simulink subsystem "LRLM_ECU_V6"  (R2021a)
settings: Solver=VariableStepAuto  StartTime=0.0  StopTime=10.0  RelTol=1e-3
libraries: LRLM x6
settings Model: Creator=Sai229  LastModifiedBy=Sai229

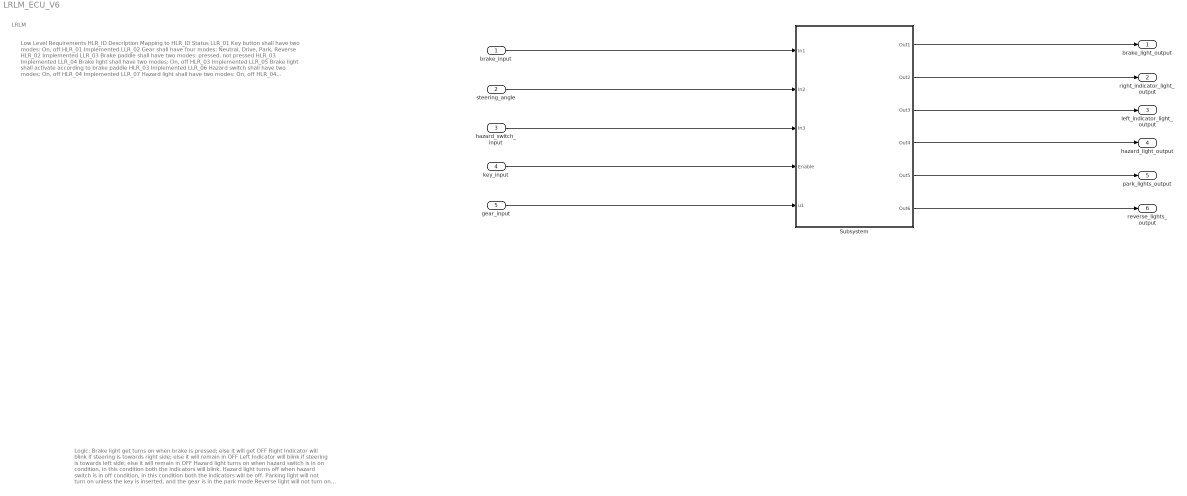
== system LRLM_ECU_V6 ==
  note: Low Level Requirements
      |
      | HLR_ID
      | Description
      | Mapping to HLR_ID
      | Status
      |
      | LLR_01
      | Key button shall have two modes: On, off
      | HLR_01
      | Implemented
      |
      | LLR_02
      | Gear shall have four modes: Neutral, Drive, Park, Reverse
      | HLR_02
      | Implemented
      |
      | LLR_03
      | Brake paddle shall have two modes: pressed, not pressed
      | HLR_03
      | Implemented
      |
      | LLR_04
      | Brake light shall have two modes: On, off
      | HLR_03
      | Implemented
      |
      | LLR_05
      | Brake light shall activate according to brake paddle
      | HLR_03
      | Implemented
      |
      | LLR_06
      | Hazard switch shall have two modes: On, off
      | HLR_04
      | Implemented
      |
      | LLR_07
      | Hazard light shall have two modes: On, off
      | HLR_04
      | Implemented
      |
      | LLR_08
      | Hazard light shall activate according to hazard switch
      | HLR_04
      | Implemented
      |
      | LLR_09
      | Steering shall move in both the directions
      | HLR_05
      | Implemented
      |
      | LLR_10
      | Right Indicator light shall have two modes: On, off
      | HLR_05
      | Implemented
      |
      | LLR_11
      | Left Indicator light shall have two modes: On, off
      | HLR_05
      | Implemented
      |
      | LLR_12
      | Right indicator light shall activate according to steering angle
      | HLR_05
      | Implemented
      |
      | LLR_13
      | Left indicator light shall activate according to steering angle
      | HLR_05
      | Implemented
      |
      | LLR_14
      | Park light shall have two modes: On, off
      | HLR_06
      | Implemented
      |
      | LLR_15
      | Parking light shall activate according to park gear and key button
      | HLR_06
      | Implemented
      |
      | LLR_16
      | Reverse light shall have two modes: On, off
      | HLR_07
      | Implemented
      |
      | LLR_17
      | Reversing lights shall activate according to reverse gear and key button
      | HLR_07
      | Implemented
  note: Logic:
      | Brake light get turns on when brake is pressed; else it will get OFF
      | Right Indicator will blink if steering is towards right side; else it will remain in OFF
      | Left Indicator will blink if steering is towards left side; else it will remain in OFF
      | Hazard light turns on when hazard switch is in on condition, in this condition both the indicators will blink.
      | Hazard light turns off when hazard switch is in off condition, in this condition both the indicators will be off.
      | Parking light will not turn on unless the key is inserted, and the gear is in the park mode
      | Reverse light will not turn on unless the key is inserted, and the gear is in the reverse mode
  note: LRLM
  brake_input : Inport
  steering_angle : Inport  Port=2
  hazard_switch_input : Inport  Port=3
  key_input : Inport  Port=4
  gear_input : Inport  Port=5
  Subsystem : Subsystem
  brake_light_output : Outport
  right_indicator_light_output : Outport  Port=2
  left_indicator_light_output : Outport  Port=3
  hazard_light_output : Outport  Port=4
  park_lights_output : Outport  Port=5
  reverse_lights_output : Outport  Port=6
  wires:
  brake_input/1 -> Subsystem/1(In1)
  steering_angle/1 -> Subsystem/2(In2)
  hazard_switch_input/1 -> Subsystem/3(In3)
  key_input/1 -> Subsystem/4(Enable)
  gear_input/1 -> Subsystem/5(u1)
  Subsystem/1(Out1) -> brake_light_output/1
  Subsystem/2(Out2) -> right_indicator_light_output/1
  Subsystem/3(Out3) -> left_indicator_light_output/1
  Subsystem/4(Out4) -> hazard_light_output/1
  Subsystem/5(Out5) -> park_lights_output/1
  Subsystem/6(Out6) -> reverse_lights_output/1

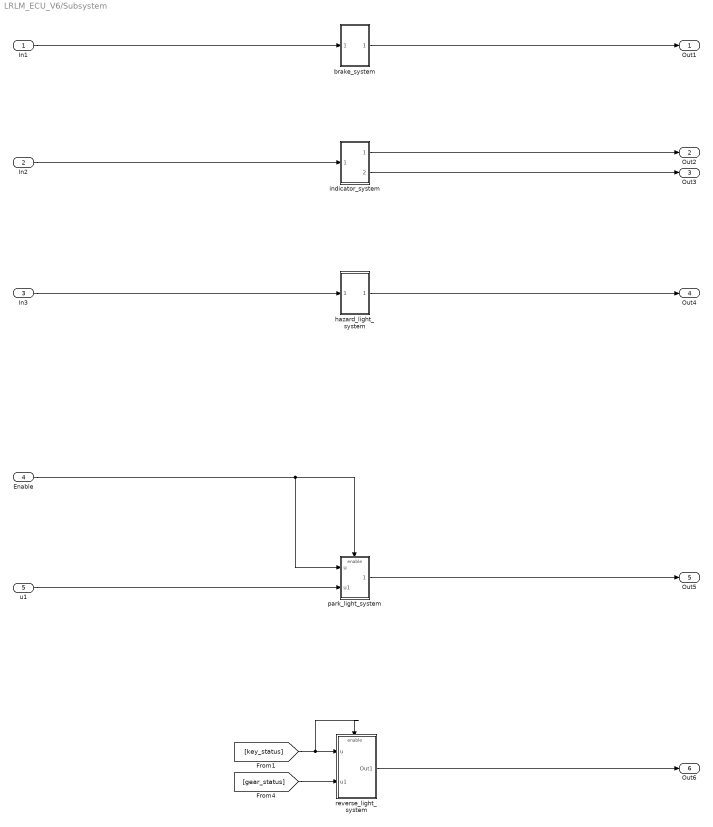
== system LRLM_ECU_V6/Subsystem ==
  In1 : Inport
  In2 : Inport  Port=2
  In3 : Inport  Port=3
  Enable : Inport  Port=4
  u1 : Inport  Port=5
  brake_system : Subsystem
  hazard_light_system : Subsystem
  indicator_system : Subsystem
  park_light_system : Subsystem
  reverse_light_system : Subsystem
  Out1 : Outport
  Out2 : Outport  Port=2
  Out3 : Outport  Port=3
  Out4 : Outport  Port=4
  Out5 : Outport  Port=5
  Out6 : Outport  Port=6
  wires:
  In3/1 -> hazard_light_system/1(In1)
  [gear_status] -> reverse_light_system/2(u1)
  hazard_light_system/1(Out1) -> Out4/1
  park_light_system/1(Out1) -> Out5/1
  [key_status] -> reverse_light_system/1(u), reverse_light_system/Enable
  Enable/1 -> park_light_system/Enable, park_light_system/1(u)
  indicator_system/2(Out2) -> Out3/1
  In2/1 -> indicator_system/1(In1)
  In1/1 -> brake_system/1(In1)
  indicator_system/1(Out1) -> Out2/1
  reverse_light_system/1(Out1) -> Out6/1
  u1/1 -> park_light_system/2(u1)
  brake_system/1(Out1) -> Out1/1

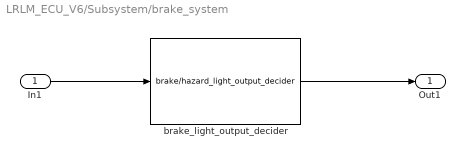
== system LRLM_ECU_V6/Subsystem/brake_system ==
  In1 : Inport
  brake_light_output_decider : LRLM/brake//hazard_light_output_decider
      settings: SourceProductName=LRLM Library
  Out1 : Outport
  wires:
  brake_light_output_decider/1 -> Out1/1
  In1/1 -> brake_light_output_decider/1

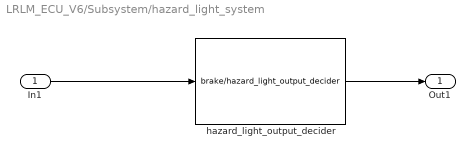
== system LRLM_ECU_V6/Subsystem/hazard_light_system ==
  In1 : Inport
  hazard_light_output_decider : LRLM/brake//hazard_light_output_decider
      settings: SourceProductName=LRLM Library
  Out1 : Outport
  wires:
  hazard_light_output_decider/1 -> Out1/1
  In1/1 -> hazard_light_output_decider/1

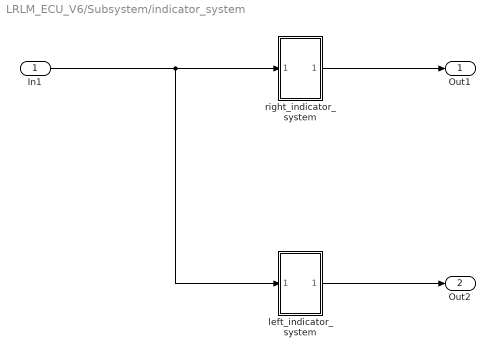
== system LRLM_ECU_V6/Subsystem/indicator_system ==
  In1 : Inport
  left_indicator_system : Subsystem
  right_indicator_system : Subsystem
  Out1 : Outport
  Out2 : Outport  Port=2
  wires:
  right_indicator_system/1(Out1) -> Out1/1
  left_indicator_system/1(Out1) -> Out2/1
  In1/1 -> right_indicator_system/1(In1), left_indicator_system/1(In1)

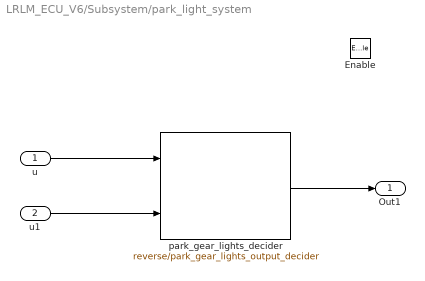
== system LRLM_ECU_V6/Subsystem/park_light_system ==
  u : Inport
  u1 : Inport  Port=2
  Enable : EnablePort  StatesWhenEnabling=reset
  park_gear_lights_decider : LRLM/reverse//park_gear_lights_output_decider  gear_option=Neutral
      settings: SourceProductName=LRLM Library
  Out1 : Outport
  wires:
  park_gear_lights_decider/1 -> Out1/1
  u1/1 -> park_gear_lights_decider/2
  u/1 -> park_gear_lights_decider/1

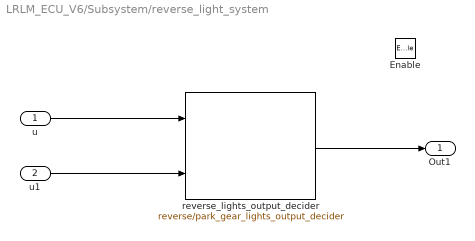
== system LRLM_ECU_V6/Subsystem/reverse_light_system ==
  u : Inport
  u1 : Inport  Port=2
  Enable : EnablePort  StatesWhenEnabling=reset
  reverse_lights_output_decider : LRLM/reverse//park_gear_lights_output_decider  gear_option=Reverse
      settings: SourceProductName=LRLM Library
  Out1 : Outport
  wires:
  reverse_lights_output_decider/1 -> Out1/1
  u1/1 -> reverse_lights_output_decider/2
  u/1 -> reverse_lights_output_decider/1

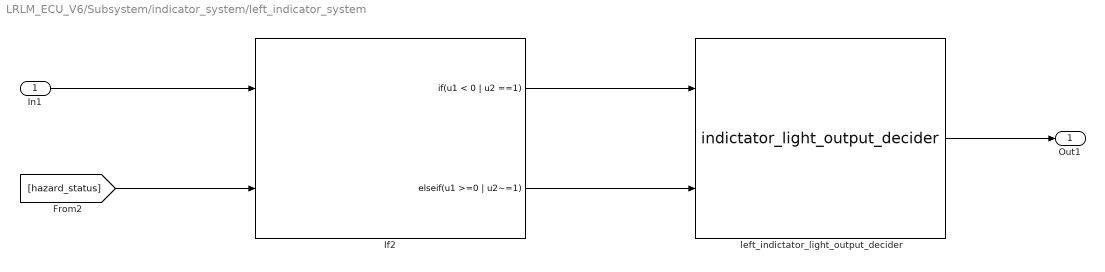
== system LRLM_ECU_V6/Subsystem/indicator_system/left_indicator_system ==
  In1 : Inport
  If2 : If  NumInputs=2  IfExpression=u1 < 0 | u2 ==1  ElseIfExpressions=u1 >=0 | u2~=1  ShowElse=off
  left_indictator_light_output_decider : LRLM/indictator_light_output_decider
      settings: SourceProductName=LRLM Library
  Out1 : Outport
  wires:
  left_indictator_light_output_decider/1 -> Out1/1
  If2/2 -> left_indictator_light_output_decider/2
  If2/1 -> left_indictator_light_output_decider/1
  In1/1 -> If2/1
  [hazard_status] -> If2/2

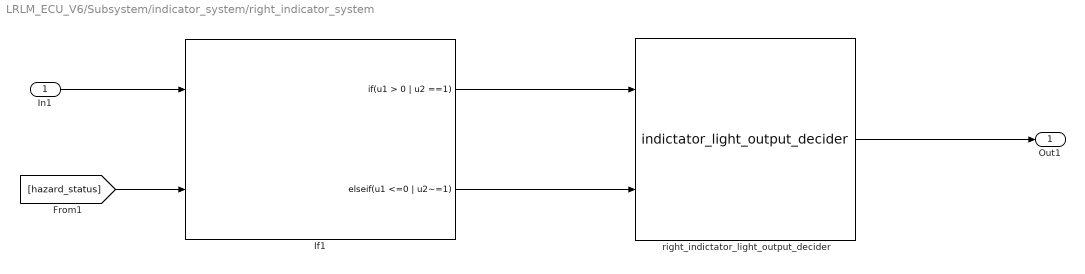
== system LRLM_ECU_V6/Subsystem/indicator_system/right_indicator_system ==
  In1 : Inport
  If1 : If  NumInputs=2  IfExpression=u1 > 0 | u2 ==1  ElseIfExpressions=u1 <=0 | u2~=1  ShowElse=off
  right_indictator_light_output_decider : LRLM/indictator_light_output_decider
      settings: SourceProductName=LRLM Library
  Out1 : Outport
  wires:
  right_indictator_light_output_decider/1 -> Out1/1
  If1/2 -> right_indictator_light_output_decider/2
  If1/1 -> right_indictator_light_output_decider/1
  In1/1 -> If1/1
  [hazard_status] -> If1/2
